simulink model "test_kinectExia"  (R2017a)
settings: Solver=VariableStepAuto  StartTime=0.0  StopTime=inf  RelTol=1e-3
undefined symbols (not defined in the file): armInitPos, BodyIndexFrame, BodyTrackingID, ColorJointIndices, DepthJointIndices, erosion, gray, HandLeftConfidence, HandLeftState, HandRightConfidence, HandRightState, IsBodyTracked, JointPositions, JointTrackingState, limit_range_ANA, limit_range_IMG, none, range_mm, relationOfArmCam, strel, value, videoinput
libraries: simulink x6, visionmorphops x3, visiontextngfix x2, imaqlib x2, visionstatistics x1, vrlib x1
settings Model: Creator=tomato  LastModifiedBy=tomato

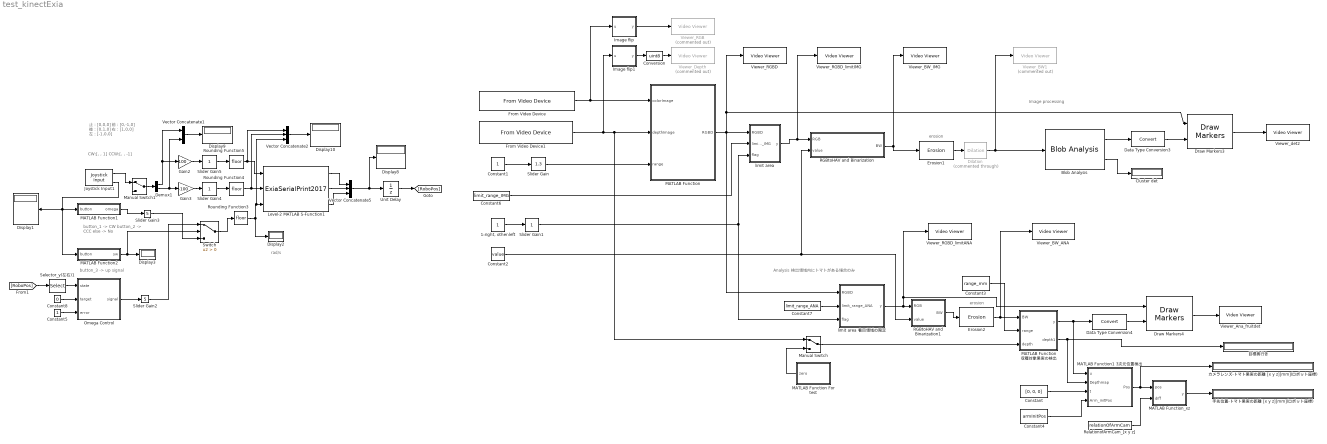
== system test_kinectExia ==
  note: erosion
  note: Image processing
  note: Analysis 検出領域内にトマトがある場合のみ
  note: erosion
  note: CW:[, , 1]
      | CCW:[, , -1]
  note: button_3 -> up signal
  note: rad/s
  note: 止：[0,0,0]
      | 前：[0,-1,0]
      | 後：[0,1,0]
      | 右：[1,0,0]
      | 左：[-1,0,0]
  note: button_1 -> CW
      | button_2 -> CCC
      | else -> No
  "1:right, other:left" : Constant
  Blob Analysis : visionstatistics/Blob Analysis  Tag=vipblks_row_conv  area=off  centroid=on  bBox=off  majorAxis=off  minorAxis=off  angle=off  eccentricity=off  equivDiameterSq=off  extent=off  perimeter=off  maxBlobs=1  warnIfNumBlobsExceeded=on  isCount=on  useMinArea=off  minArea=0  useMaxArea=off  maxArea=intmax('uint32')  excludeBorderBlob=off  outDT=double  isOutVarDim=off  isFill=on  fillValues=-1  conn=8  isLabel=off  outputMode=Binary point scaling  outputWordLength=32  outputFracLength=16  firstCoeffMode=Binary point scaling  firstCoeffWordLength=16  firstCoeffFracLength=14  secondCoeffMode=Binary point scaling  secondCoeffWordLength=32  secondCoeffFracLength=16  accumMode=Binary point scaling  accumWordLength=32  accumFracLength=0  prodOutputMode=Binary point scaling  prodOutputWordLength=32  prodOutputFracLength=16  roundingMode=Floor  overflowMode=off
      settings: SourceProductName=Computer Vision System Toolbox
  Cluster det : Display
  Constant : Constant  Value=[0, 0, 0]
  Constant1 : Constant
  Constant2 : Constant  Value=value
  Constant3 : Constant  Value=range_mm
  Constant4 : Constant  Value=armInitPos
  Constant5 : Constant
  Constant6 : Constant  Value=limit_range_IMG
  Constant7 : Constant  Value=limit_range_ANA
  Constant8 : Constant  Value=0
  Conversion : DataTypeConversion  OutDataTypeStr=uint8
  Data Type Conversion3 : DataTypeConversion
  Data Type Conversion4 : DataTypeConversion
  Demux1 : Demux  Outputs=2
  Dilation : visionmorphops/Dilation  Commented=through  nhoodsrc=Specify via dialog  strel=strel('disk',1)
      settings: SourceProductName=Computer Vision System Toolbox  SourceProductBaseCode=VP
  Display{1..3,8..10} (6 alike) : Display
  Draw Markers3 : visiontextngfix/Draw Markers  shape=Circle  size=5  fill=on  fillClrSource=Specify via dialog  display=User-specified value  intensity=200  color=[0 0 255]  opacity=0.6  viewport=Entire image  antialiasing=off  inType=Obsolete  imagePorts=One multidimensional signal  prodOutputMode=Binary point scaling  prodOutputWordLength=32  prodOutputFracLength=14  memoryMode=Specify word length  memoryWordLength=16  memoryFracLength=14  roundingMode=Floor  overflowMode=off
      settings: SourceProductName=Computer Vision System Toolbox  SourceProductBaseCode=VP
  Draw Markers4 : visiontextngfix/Draw Markers  shape=Circle  size=5  fill=on  fillClrSource=Specify via dialog  display=User-specified value  intensity=200  color=[0 0 255]  opacity=0.6  viewport=Entire image  antialiasing=off  inType=Obsolete  imagePorts=One multidimensional signal  prodOutputMode=Binary point scaling  prodOutputWordLength=32  prodOutputFracLength=14  memoryMode=Specify word length  memoryWordLength=16  memoryFracLength=14  roundingMode=Floor  overflowMode=off
      settings: SourceProductName=Computer Vision System Toolbox  SourceProductBaseCode=VP
  Erosion1 : visionmorphops/Erosion  nhoodsrc=Specify via dialog  strel=strel('disk',erosion)
      settings: SourceProductName=Computer Vision System Toolbox  SourceProductBaseCode=VP
  Erosion2 : visionmorphops/Erosion  nhoodsrc=Specify via dialog  strel=strel('disk',erosion)
      settings: SourceProductName=Computer Vision System Toolbox  SourceProductBaseCode=VP
  From Video Device : imaqlib/From Video Device  DeviceMenu=kinect 1 (Kinect V2 Color Sensor)  Device=kinect 1 (Kinect V2 Color Sensor)  ObjConstructor=videoinput('kinect', 1)  VideoFormatMenu=MJPG_1280x720  VideoFormat=BGR_1920x1080  VideoSource=Kinect V2 Color Source  ROIPosition=[0 0 1080 1920]  EnableHWTrigger=off  TriggerConfiguration=kinect 1 (Kinect V2 Color Sensor)  SampleTime=0.3  OutputPortsMode=One multidimensional signal  DataType=uint8  CanDoHWTrigger=no  ReturnedColorSpace=rgb  BlockHandle=6.0001  ROIWidth=1920  ROIHeight=1080  ROIColumn=0  ROIRow=0  EngXMLPath=C:\Program Files\MATLAB\R2017a\toolbox\imaq\imaq\private  DevXMLPath=C:\ProgramData\MATLAB\SupportPackages\R2017a\toolbox\imaq\supportpackages\kinectruntime\adaptor\win64  EngLibPath=C:\Program Files\MATLAB\R2017a\toolbox\imaq\imaqblks\imaqmex\win64  ColorSpace=rgb  BayerSensorAlignment=grbg
      settings: SourceProductName=Image Acquisition Toolbox
  From Video Device1 : imaqlib/From Video Device  DeviceMenu=kinect 1 (Kinect V2 Color Sensor)  Device=kinect 2 (Kinect V2 Depth Sensor)  ObjConstructor=videoinput('kinect', 2)  VideoFormatMenu=MJPG_1280x720  VideoFormat=Depth_512x424  VideoSource=Kinect V2 Depth Source  ROIPosition=[0 0 424 512]  EnableHWTrigger=off  TriggerConfiguration=none/none  SampleTime=0.3  OutputPortsMode=One multidimensional signal  DataType=uint16  CanDoHWTrigger=no  ReturnedColorSpace=grayscale  BlockHandle=6.0001  ROIWidth=512  ROIHeight=424  ROIColumn=0  ROIRow=0  EngXMLPath=C:\Program Files\MATLAB\R2017a\toolbox\imaq\imaq\private  DevXMLPath=C:\ProgramData\MATLAB\SupportPackages\R2017a\toolbox\imaq\supportpackages\kinectruntime\adaptor\win64  EngLibPath=C:\Program Files\MATLAB\R2017a\toolbox\imaq\imaqblks\imaqmex\win64  ColorSpace=grayscale  BayerSensorAlignment=grbg  AllMetadata=BodyIndexFrame;BodyTrackingID;ColorJointIndices;DepthJointIndices;HandLeftConfidence;HandLeftState;HandRightConfidence;HandRightState;IsBodyTracked;JointPositions;JointTrackingState
      settings: SourceProductName=Image Acquisition Toolbox
  Gain2 : Gain  Gain=100
  Gain3 : Gain  Gain=-100
  Image flip : MATLAB Function  TreatAsAtomicUnit=on
  Image flip1 : MATLAB Function  TreatAsAtomicUnit=on
  Joystick Input1 : vrlib/Joystick Input  joyid=1  adjustports=on  forcefeed=off
      settings: SourceProductBaseCode=VR
  Level-2 MATLAB S-Function1 : M-S-Function  FunctionName=ExiaSerialPrint2017  Parameters='COM13'
  MATLAB Function : MATLAB Function  TreatAsAtomicUnit=on
  MATLAB Function For test : MATLAB Function  TreatAsAtomicUnit=on
  MATLAB Function 収穫対象果実の検出 : MATLAB Function  TreatAsAtomicUnit=on
  MATLAB Function1 : MATLAB Function  TreatAsAtomicUnit=on
  MATLAB Function1 3次元位置検出 : MATLAB Function  TreatAsAtomicUnit=on
  MATLAB Function2 : MATLAB Function  TreatAsAtomicUnit=on
  MATLAB Function_xz : MATLAB Function  TreatAsAtomicUnit=on
  Manual Switch : ManualSwitch
  Manual Switch1 : ManualSwitch
  Omega Control : MATLAB Function  TreatAsAtomicUnit=on
  RGBtoHAV and Binarization : MATLAB Function  TreatAsAtomicUnit=on
  RGBtoHAV and Binarization1 : MATLAB Function  TreatAsAtomicUnit=on
  RelationofArmCam_[x y z] : Constant  Value=relationOfArmCam
  Rounding Function3 : Rounding
  Rounding Function4 : Rounding
  Rounding Function5 : Rounding
  Selector_y(左右)1 : Selector  InputPortWidth=3  IndexOptions=Index vector (dialog)  Indices=3  OutputSizes=1
  Slider Gain : simulink/Math Operations/Slider Gain  gain=1.3  low=0  high=8
  Slider Gain1 : simulink/Math Operations/Slider Gain  gain=1  low=0  high=2
  Slider Gain2 : simulink/Math Operations/Slider Gain  gain=5  low=-10  high=10
  Slider Gain3 : simulink/Math Operations/Slider Gain  gain=5  low=-10  high=10
  Slider Gain4 : simulink/Math Operations/Slider Gain  gain=1  low=-4  high=10
  Slider Gain5 : simulink/Math Operations/Slider Gain  gain=1  low=-5  high=10
  Switch : Switch  Criteria=u2 > Threshold
  Unit Delay : UnitDelay  SampleTime=-1
  Vector Concatenate1 : Concatenate
  Vector Concatenate2 : Concatenate  NumInputs=3
  Vector Concatenate5 : Concatenate  NumInputs=3
  Viewer_Ana_fruitdet : VideoViewer  colormapValue=gray(256)  FigPos=[1514 544 396 330]
  Viewer_BW1 : VideoViewer  Commented=on  colormapValue=gray(256)  FigPos=[685 929 418 304]
  Viewer_BW_ANA : VideoViewer  colormapValue=gray(256)  FigPos=[1379 1090 418 304]
  Viewer_BW_IMG : VideoViewer  colormapValue=gray(256)  FigPos=[650 424 418 304]
  Viewer_Depth : VideoViewer  Commented=on  colormapValue=gray(256)  FigPos=[326 827 418 304]
  Viewer_RGB : VideoViewer  Commented=on  colormapValue=gray(256)  FigPos=[119 580 418 301]
  Viewer_RGBD : VideoViewer  colormapValue=gray(256)  FigPos=[1186 523 418 304]
  Viewer_RGBD_limitANA : VideoViewer  colormapValue=gray(256)  FigPos=[729 882 418 304]
  Viewer_RGBD_limitIMG : VideoViewer  colormapValue=gray(256)  FigPos=[197 459 418 307]
  Viewer_det2 : VideoViewer  colormapValue=gray(256)  FigPos=[938 457 418 304]
  limit area : MATLAB Function  TreatAsAtomicUnit=on
  limit area 着目領域の限定 : MATLAB Function  TreatAsAtomicUnit=on
  カメラレンズ-トマト果実の距離 [x y z][mm](ロボット座標) : Display
  手先位置-トマト果実の距離 [x y z][mm](ロボット座標) : Display
  目標奥行き : Display
  wires:
  RGBtoHAV and Binarization/1(BW) -> Erosion1/1, Viewer_BW_IMG/1
  Erosion1/1 -> Dilation/1
  From Video Device/1 -> Image flip/1(u), MATLAB Function/1(colorImage)
  Constant1/1 -> Slider Gain/1
  Slider Gain/1 -> MATLAB Function/3(range)
  limit area/1(y) -> RGBtoHAV and Binarization/1(RGB), Viewer_RGBD_limitIMG/1
  "1:right, other:left"/1 -> Slider Gain1/1
  Slider Gain1/1 -> limit area 着目領域の限定/3(flag), limit area/3(flag)
  Blob Analysis/1 -> Data Type Conversion3/1
  Conversion/1 -> Viewer_Depth/1
  Image flip1/1(y) -> Conversion/1
  Draw Markers3/1 -> Viewer_det2/1
  Data Type Conversion3/1 -> Draw Markers3/2
  Dilation/1 -> Viewer_BW1/1, Blob Analysis/1
  MATLAB Function 収穫対象果実の検出/1(y) -> MATLAB Function1 3次元位置検出/1(u), Data Type Conversion4/1
  Draw Markers4/1 -> Viewer_Ana_fruitdet/1
  Data Type Conversion4/1 -> Draw Markers4/2
  Blob Analysis/2 -> Cluster det/1
  MATLAB Function/1(RGBD) -> limit area/1(RGBD), Viewer_RGBD/1, Draw Markers3/1, limit area 着目領域の限定/1(RGBD)
  Constant2/1 -> RGBtoHAV and Binarization1/2(value), RGBtoHAV and Binarization/2(value)
  Image flip/1(y) -> Viewer_RGB/1
  MATLAB Function_xz/1(y) -> 手先位置-トマト果実の距離 [x y z][mm](ロボット座標)/1
  MATLAB Function 収穫対象果実の検出/2(depth1) -> MATLAB Function1 3次元位置検出/2(Depthmap), 目標奥行き/1
  From Video Device1/1 -> Manual Switch/1, MATLAB Function/2(depthImage), Image flip1/1(u)
  MATLAB Function1 3次元位置検出/1(Pos) -> カメラレンズ-トマト果実の距離 [x y z][mm](ロボット座標)/1, MATLAB Function_xz/1(pos)
  Constant6/1 -> limit area/2(limit_range_IMG)
  Constant7/1 -> limit area 着目領域の限定/2(limit_range_ANA)
  RGBtoHAV and Binarization1/1(BW) -> Erosion2/1
  Constant3/1 -> MATLAB Function 収穫対象果実の検出/2(range)
  MATLAB Function For test/1(zero) -> Manual Switch/2
  Manual Switch/1 -> MATLAB Function 収穫対象果実の検出/3(depth)
  Constant/1 -> MATLAB Function1 3次元位置検出/3(t)
  Constant4/1 -> MATLAB Function1 3次元位置検出/4(Arm_initPos)
  RelationofArmCam_[x y z]/1 -> MATLAB Function_xz/2(diff)
  limit area 着目領域の限定/1(y) -> Viewer_RGBD_limitANA/1, Draw Markers4/1, RGBtoHAV and Binarization1/1(RGB)
  Erosion2/1 -> Viewer_BW_ANA/1, MATLAB Function 収穫対象果実の検出/1(BW)
  Constant5/1 -> Omega Control/3(error)
  Switch/1 -> Rounding Function3/1
  Gain2/1 -> Slider Gain5/1
  Level-2 MATLAB S-Function1/1 -> Vector Concatenate5/1
  Unit Delay/1 -> [RoboPos]
  [RoboPos] -> Selector_y(左右)1/1
  Demux1/1 -> Vector Concatenate1/1, Gain2/1
  MATLAB Function1/1(omega) -> Slider Gain3/1
  Level-2 MATLAB S-Function1/3 -> Vector Concatenate5/3
  Rounding Function5/1 -> Vector Concatenate2/1, Level-2 MATLAB S-Function1/1
  Slider Gain3/1 -> Switch/3
  Slider Gain5/1 -> Rounding Function5/1
  Rounding Function4/1 -> Vector Concatenate2/2, Level-2 MATLAB S-Function1/2
  Gain3/1 -> Slider Gain4/1
  Vector Concatenate5/1 -> Unit Delay/1, Display8/1
  Slider Gain4/1 -> Rounding Function4/1
  Demux1/2 -> Vector Concatenate1/2, Gain3/1
  Vector Concatenate2/1 -> Display10/1
  Manual Switch1/1 -> Demux1/1
  Slider Gain2/1 -> Switch/1
  Selector_y(左右)1/1 -> Omega Control/1(state)
  Rounding Function3/1 -> Display2/1, Vector Concatenate2/3, Level-2 MATLAB S-Function1/3
  MATLAB Function2/1(sw) -> Switch/2, Display3/1
  Level-2 MATLAB S-Function1/2 -> Vector Concatenate5/2
  Joystick Input1/2 -> MATLAB Function2/1(button), MATLAB Function1/1(button), Display1/1
  Omega Control/1(signal) -> Slider Gain2/1
  Joystick Input1/1 -> Manual Switch1/1
  Vector Concatenate1/1 -> Display9/1
  Constant8/1 -> Omega Control/2(target)

== matlab function test_kinectExia/MATLAB Function For test ==
  data: zero output
function zero = fcn()
zero = zeros(424,512);

== matlab function test_kinectExia/RGBtoHAV and Binarization ==
  data: RGB input; BW output; value input
function BW = createMask(RGB, value)
%createMask  Threshold RGB image using auto-generated code from colorThresholder app.
%  [BW,MASKEDRGBIMAGE] = createMask(RGB) thresholds image RGB using
%  auto-generated code from the colorThresholder App. The colorspace and
%  minimum/maximum values for each channel of the colorspace were set in the
%  App and result in a binary mask BW and a composite image maskedRGBImage,
%  which shows the original RGB image values under the mask BW.

% Auto-generated by colorThresholder app on 12-Apr-2017
%------------------------------------------------------


% Convert RGB image to chosen color space
I = rgb2hsv(RGB);
%%
% H
channel1Min = value(1);
channel1Max = value(2);
% S
channel2Min = value(3);
channel2Max = value(4);
% V
channel3Min = value(5);
channel3Max = value(6);

% Create mask based on chosen histogram thresholds
sliderBW = ( (I(:,:,1) >= channel1Min) | (I(:,:,1) <= channel1Max) ) & ...
    (I(:,:,2) >= channel2Min ) & (I(:,:,2) <= channel2Max) & ...
    (I(:,:,3) >= channel3Min ) & (I(:,:,3) <= channel3Max);
%%
BW = sliderBW;

end

== matlab function test_kinectExia/Image flip1 ==
  data: u input; y output
function y = fcn(u)

y = fliplr(u);

== matlab function test_kinectExia/Image flip ==
  data: u input; y output
function y = fcn(u)

y = fliplr(u);

== matlab function test_kinectExia/MATLAB Function 収穫対象果実の検出 ==
  data: BW input; range input; y output; depth input; depth1 output
function [y,depth1] = fcn(BW,range, depth)
y = [0, 0];
depth = fliplr(depth);
depth1 = 0;
% %% 非ゼロ検出
[row,col] = find(BW);
 s=size(row);
 n=s(1);
 if n ~= 0
    position=zeros(n,3);
    for i=1:n
        position(i,1)=col(i);
        position(i,2)=row(i);
        position(i,3)=depth(row(i), col(i));
    end
%%
    [row2,col2, v] = find(position(:,3));

    [M, Index]=min(v);

    a=0;b=0;
    a=position(row2(Index),1);
    b=position(row2(Index),2);

    disp(position(row2(Index),1))
%%
    Dav = uint16(0);
    count = 0;
    for i = -1: 1
        for j = -1: 1
            if (BW(b + j, a + i) == 1) && (depth(b + j, a + i) ~= 0) && (depth(b + j, a + i) <= range)
                Dav = Dav + depth(b + j, a + i);
                count = count + 1;
                disp(depth(b + j, a + i));
            end
        end
    end
    Dav = Dav / count;

    if Dav == 0
        Dav = uint16(670);
    end

    y = [a, b];
    depth1 = double(Dav);
 end

== matlab function test_kinectExia/RGBtoHAV and Binarization1 ==
  data: RGB input; BW output; value input
function BW = createMask(RGB, value)
%createMask  Threshold RGB image using auto-generated code from colorThresholder app.
%  [BW,MASKEDRGBIMAGE] = createMask(RGB) thresholds image RGB using
%  auto-generated code from the colorThresholder App. The colorspace and
%  minimum/maximum values for each channel of the colorspace were set in the
%  App and result in a binary mask BW and a composite image maskedRGBImage,
%  which shows the original RGB image values under the mask BW.

% Auto-generated by colorThresholder app on 12-Apr-2017
%------------------------------------------------------


% Convert RGB image to chosen color space
I = rgb2hsv(RGB);
%%
% H
channel1Min = value(1);
channel1Max = value(2);
% S
channel2Min = value(3);
channel2Max = value(4);
% V
channel3Min = value(5);
channel3Max = value(6);

% Create mask based on chosen histogram thresholds
sliderBW = ( (I(:,:,1) >= channel1Min) | (I(:,:,1) <= channel1Max) ) & ...
    (I(:,:,2) >= channel2Min ) & (I(:,:,2) <= channel2Max) & ...
    (I(:,:,3) >= channel3Min ) & (I(:,:,3) <= channel3Max);
%%
BW = sliderBW;

end

== matlab function test_kinectExia/MATLAB Function_xz ==
  data: pos input; y output; diff input
function y = fcn(pos,diff)
y=[0, 0, 0];
% [x, y, z](Arm座標)
% x

% 直線距離の算出
pos(1)=pos(1)*cos(asin((pos(2))/pos(1)));


y(1) = pos(1) - diff(1); 
% y
y(2) = diff(2)-pos(2);
% z
%y(3) = diff(3)-pos(3);
y(3) = pos(3) - diff(3);

== matlab function test_kinectExia/MATLAB Function1 ==
  data: button input; omega output
function omega = fcn(button)

% CW
if button(1) == 1
    omega = -1;
% CCW
elseif button(2) == 1
    omega = 1;
else
    omega = 0;
end

== matlab function test_kinectExia/MATLAB Function1 3次元位置検出 ==
  data: u input; Pos output; Depthmap input; t input; Arm_initPos input
function Pos = fcn(u, Depthmap, t ,Arm_initPos)

Pos = [u(1), u(2), -1];
%Depthmap=fliplr(Depthmap);

coder.extrinsic('evalin', 'pointsToWorld')
Params = evalin('base', 'IRcameraParams');
R = evalin('base', 'R');
% t = evalin('base', 't');

if u(2)~=-1 && Depthmap ~= 0
    %ArmX=double(Depthmap(round(u(2)), round(u(1))));
    ArmX=double(Depthmap);
    t(3)=ArmX;
    imagePoints=[u(1), u(2)];

    % 画像座標を世界座標へ
    worldPoints1 = pointsToWorld(Params, R, t, imagePoints);
    % disp(worldPoints1(1));
    % disp(worldPoints1(2));
    ArmY=worldPoints1(1);
    ArmZ=worldPoints1(2);
    %test = round(ArmY) - 80; 
    
    Pos = [ArmX, ArmY, ArmZ];
    Pos(3) = -1 * ArmZ;     % -1をかける
    Pos(2) = Pos(2) -80;    % kinectのずれ補正
else
    Pos = [Arm_initPos(1),Arm_initPos(2), Arm_initPos(3)];
end

== matlab function test_kinectExia/MATLAB Function2 ==
  data: button input; sw output
function sw = fcn(button)

if button(3) == 1
    sw = 1;
else
    sw =0;
end

== matlab function test_kinectExia/MATLAB Function ==
  data: colorImage input; RGBD output uint8 size=[424 512 3]; depthImage input; range input
function RGBD  = fcn(colorImage, depthImage, range)

coder.extrinsic('pcfromkinect')
coder.extrinsic('evalin')
coder.extrinsic('getfield')

device = evalin('base', 'depthDevice');

pc = pcfromkinect(device,depthImage,colorImage, 'depthCentric');
a = single(zeros(424, 512,3));
b = uint8(zeros(424, 512,3));
a = getfield(pc, 'Location');
b = getfield(pc, 'Color');

for i=1:424
   for j=1:512
       if a(i,j,3) < range
           b(i,j,:)=b(i,j,:);
       else
           b(i,j,:)=255;
       end
   end
end

RGBD=b;

% y = single(zeros(424, 512));
% y = fliplr(getfield(pc, 'Location'));
% y = fliplr(y);

== matlab function test_kinectExia/Omega Control ==
  data: state input; target input; error input; signal output
function signal = fcn(state, target, error)

% CCW補正(左回転)
if state > target + error
    signal = -1;
% CW補正(右回転)
elseif state < target -1 * error
    signal = 1;
else
    signal = 0;
end

== matlab function test_kinectExia/limit area 着目領域の限定 ==
  data: RGBD input; y output; limit_range_ANA input; flag input
function y = fcn(RGBD, limit_range_ANA, flag)

% 上側除去
for i=1:limit_range_ANA(1)
    RGBD(i,:,:)=0;
end
% 下側除去
for i=limit_range_ANA(2):424
    RGBD(i,:,:)=0;
end

% 424*512pixel
% 横半分256の半分128±50pixel
% 右側着目：flag = 1 : 左側領域除去：i=78:178
% 左側着目：other    : 右側領域除去：i=334:438
    
if flag==1
    % 左側除去
    for i=1:limit_range_ANA(3)
        RGBD(:,i,:)=0;
    end
    for i=limit_range_ANA(4):512
        RGBD(:,i,:)=0;
    end
else
    % 右側除去
    for i=1:limit_range_ANA(5)
        RGBD(:,i,:)=0;
    end
    for i=limit_range_ANA(6):512
        RGBD(:,i,:)=0;
    end
end

y=RGBD;

== matlab function test_kinectExia/limit area ==
  data: RGBD input; y output; limit_range_IMG input; flag input
function y = fcn(RGBD, limit_range_IMG, flag)

% 上半分除去
for i=1:limit_range_IMG(1)
    RGBD(i,:,:)=0;
end

for i=limit_range_IMG(2):424
    RGBD(i,:,:)=0;
end

% 424*512pixel
% 横半分256の半分128±50pixel
% u(:,i,:)=
% 左側領域：i=78:178
% 右側領域：i=334:438
    
if flag==1
    % 左側除去
    for i=1:limit_range_IMG(3)
        RGBD(:,i,:)=0;
    end
    for i=limit_range_IMG(4):512
        RGBD(:,i,:)=0;
    end
else
    % 右側除去
    for i=1:limit_range_IMG(5)
        RGBD(:,i,:)=0;
    end
    for i=limit_range_IMG(6):512
        RGBD(:,i,:)=0;
    end
end

y=RGBD;
